simulink library "lib_Deformation_ThermExp1DElastic"  (R2015a)
settings: Solver=ode45  StartTime=0.0  StopTime=10.0  RelTol=1e-3
settings Model: Creator=jlkratz  LastModifiedBy=jlkratz

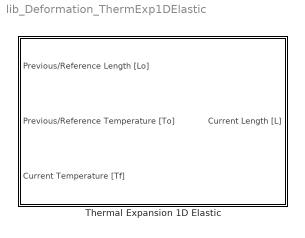
== system lib_Deformation_ThermExp1DElastic ==
  Thermal Expansion 1D Elastic : Subsystem  mask(TSAT: Thermal Expansion Library Block){TempDependence_M=on, alpha_M=0.000001, T_data_M=[500 1000], alpha_data_M=[0.000001 0.000001], BN_M=double(gcb)}
      mask prompts: TempDependence_M "TempDependence_M - Temperature dependence of the thermal expansion coefficient (unchecked - constant, checked - temperature dependent)"; alpha_M "alpha_M - Constant thermal expansion coefficient"; T_data_M "T_data_M - Temperature array (nx1)"; alpha_data_M "alpha_data_M - Thermal expansion coefficient array (nx1)"; BN_M "Block Name"
      mask help:
      | This function calculates the length or radius of a structure that has expanded or contracted due to thermal expansion. The block accepts the previous/reference length (Lo), previous/reference temperature (To), and current temperature (Tf) as its inputs. The user has the option to specify a constant thermal expansion coefficient or to incorporate temperature dependence by providing data that correlates the thermal expansion coefficient with temperature.
      |
      | This block is capable of accepting various units but it is important that the units be consistent across all inputs and parameters. For details on this block, see the block help menu.
      mask init:
      | %set default parameters if they are not being used
      | if TempDependence_M == 0
      |     T_data_M = [0 5000];
      |     alpha_data_M = [10e-6 10e-6];
      | elseif TempDependence_M == 1
      |     alpha_M = 10e-6;
      | end
      mask Help: web(which('Deformation_TSAT_ThermExp1DElastic.html'),'-helpbrowser')
      mask Callback TempDependence_M:
      | MSK_SEC_Enables_TSAT('TempDependence_M',2,'dis')
      | MSK_SEC_Enables_TSAT('TempDependence_M',[3 4],'en')

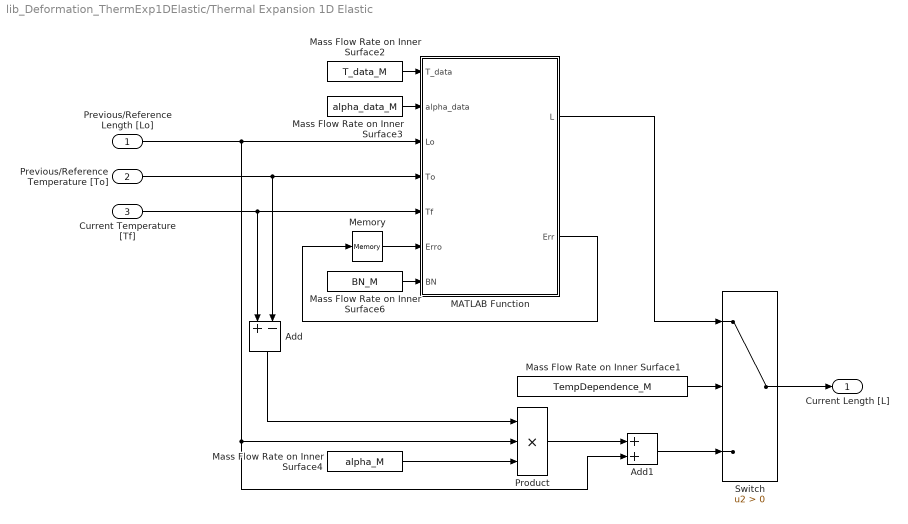
== system lib_Deformation_ThermExp1DElastic/Thermal Expansion 1D Elastic ==
  Previous/Reference Length [Lo] : Inport
  Previous/Reference Temperature [To] : Inport  Port=2
  Current Temperature [Tf] : Inport  Port=3
  Add : Sum  Inputs=+-
  Add1 : Sum
  MATLAB Function : MATLAB Function  TreatAsAtomicUnit=on
  Mass Flow Rate on Inner Surface1 : Constant  Value=TempDependence_M
  Mass Flow Rate on Inner Surface2 : Constant  Value=T_data_M
  Mass Flow Rate on Inner Surface3 : Constant  Value=alpha_data_M
  Mass Flow Rate on Inner Surface4 : Constant  Value=alpha_M
  Mass Flow Rate on Inner Surface6 : Constant  Value=BN_M
  Memory : Memory  X0=zeros(1,7)  InheritSampleTime=on
  Product : Product  Inputs=***
  Switch : Switch  Criteria=u2 > Threshold
  Current Length [L] : Outport
  wires:
  Add1/1 -> Switch/3
  Product/1 -> Add1/1
  Switch/1 -> Current Length [L]/1
  Mass Flow Rate on Inner Surface4/1 -> Product/3
  Add/1 -> Product/1
  Mass Flow Rate on Inner Surface3/1 -> MATLAB Function/2(alpha_data)
  Mass Flow Rate on Inner Surface2/1 -> MATLAB Function/1(T_data)
  Mass Flow Rate on Inner Surface1/1 -> Switch/2
  MATLAB Function/2(Err) -> Memory/1
  Memory/1 -> MATLAB Function/6(Erro)
  MATLAB Function/1(L) -> Switch/1
  Mass Flow Rate on Inner Surface6/1 -> MATLAB Function/7(BN)
  Current Temperature [Tf]/1 -> Add/1, MATLAB Function/5(Tf)
  Previous/Reference Temperature [To]/1 -> Add/2, MATLAB Function/4(To)
  Previous/Reference Length [Lo]/1 -> MATLAB Function/3(Lo), Add1/2, Product/2

== matlab function lib_Deformation_ThermExp1DElastic/Thermal Expansion 1D Elastic/MATLAB Function ==
  data: T_data input; L output; alpha_data input; Lo input; To input; Tf input; Erro input; BN input; Err output
function [L,Err] = ThermalExpansion(T_data,alpha_data,Lo,To,Tf,Erro,BN)
%#codegen

% initialize error/warning array
Err = Erro;
ErrNum = 1; %Error index

% number of data points for interpolation and numerical integration
n = 50;

%check input sizes
if length(T_data) < 2 && Erro(ErrNum) == 0
    Err(ErrNum) = 1;
    fprintf('warning in %s: The temperature data array (T_data) must be an array of at least 2 elements\n',char(BN));
end
ErrNum = ErrNum + 1;
if length(T_data) ~= length(alpha_data) && Erro(ErrNum) == 0
    Err(ErrNum) = 1;
    fprintf('warning in %s: The temperature data array (T_data) and corresponding thermal expansion coefficient data array (alpha_data) must be the same size\n',char(BN));
end
ErrNum = ErrNum + 1;
    
%check that To and Tf are in the range of T_data
if To < min(T_data)
    To = min(T_data);
    Err(ErrNum) = 1;
    if Erro(ErrNum) == 0
        fprintf('warning in %s: The previous/reference temperature (To) is less than the minimum value of the temperature data array T_data. Expand the data arrays to assure good results. The previous/reference temperature (To) has been set to the minimum value of T_data to avoid errors.\n',char(BN));
    end
end
ErrNum = ErrNum + 1;
if To > max(T_data)
    To = max(T_data);
    Err(ErrNum) = 1;
    if Erro(ErrNum) == 0
        fprintf('warning in %s: The previous/reference temperature (To) is greater than the maximum value of the temperature data array T_data. Expand the data arrays to assure good results. The previous/reference temperature (To) has been set to the maximum value of T_data to avoid errors.\n',char(BN));
    end
end
ErrNum = ErrNum + 1;
if Tf < min(T_data)
    Tf = min(T_data);
    Err(ErrNum) = 1;
    if Erro(ErrNum) == 0
        fprintf('warning in %s: The current temperature (Tf) is less than the minimum value of the temperature data array T_data. Expand the data arrays to assure good results. The current temperature (Tf) has been set to the maximum value of T_data to avoid errors.\n',char(BN));
    end
end
ErrNum = ErrNum + 1;
if Tf > max(T_data)
    Tf = max(T_data);
    Err(ErrNum) = 1;
    if Erro(ErrNum) == 0
        fprintf('warning in %s: The current temperature (Tf) is greater than the maximum value of the temperature data array T_data. Expand the data arrays to assure good results. The current temperature (Tf) has been set to the maximum value of T_data to avoid errors.\n',char(BN));
    end
end
ErrNum = ErrNum + 1;

%check that T_data is monotonically increasing
diffT = diff(T_data);
if min(diffT) <= 0 && Erro(ErrNum) == 0
    Err(ErrNum) = 1;
    fprintf('warning in %s: The temperature data array (T_data) must be monotonically increasing\n',char(BN));
end

T = linspace(To,Tf,n);
alpha = zeros(1,n);
for i = 1:n
    alpha(i) = interp1(T_data,alpha_data,T(i),'linear');
end

Int_alphadT = trapz(T,alpha);
dL = Lo*Int_alphadT;

L = Lo + dL;
